simulink model "kinematic_control"  (R2018b)
settings: Solver=FixedStepAuto  StartTime=0.0  StopTime=15  FixedStep=0.001  RelTol=1e-3
values from neighbouring files (symbols this model uses):
  Cm = 0    [kinematic_parameter.m]
  Friction = 0    [kinematic_parameter.m]
  Iyw = mw*R^2/2    (= 0.0005)    [kinematic_parameter.m]
  Izb = 1/12*(d^2+w^2)    (= 0.0433333333333)    [kinematic_parameter.m]
  Izw = mw*(lx^2+ly^2)    (= 0.045487444)    [kinematic_parameter.m]
  Jm = 0    [kinematic_parameter.m]
  Kb = Kt    (= 0.0286)    [kinematic_parameter.m]
  Kf = 0    [kinematic_parameter.m]
  Ki_deg = 3    [kinematic_parameter.m]
  Ki_m = 3    [kinematic_parameter.m]
  Ki_pos = 5    [kinematic_parameter.m]
  Kp_deg = 2    [kinematic_parameter.m]
  Kp_m = 0.5    [kinematic_parameter.m]
  Kp_pos = 3    [kinematic_parameter.m]
  Kt = 28.6*10^-3    (= 0.0286)    [kinematic_parameter.m]
  La = 0.39*10^-3    (= 0.00039)    [kinematic_parameter.m]
  lx = 0.2375    [kinematic_parameter.m]
  ly = 0.2394    [kinematic_parameter.m]
  mb = 30    [kinematic_parameter.m]
  mw = 0.4    [kinematic_parameter.m]
  N = N_motor * N_wheel    (= 14)    [kinematic_parameter.m]
  R = 0.05    [kinematic_parameter.m]
  Ra = 0.38    [kinematic_parameter.m]
libraries: simulink x1
settings Model: Creator=HONG  LastModifiedBy=HONG

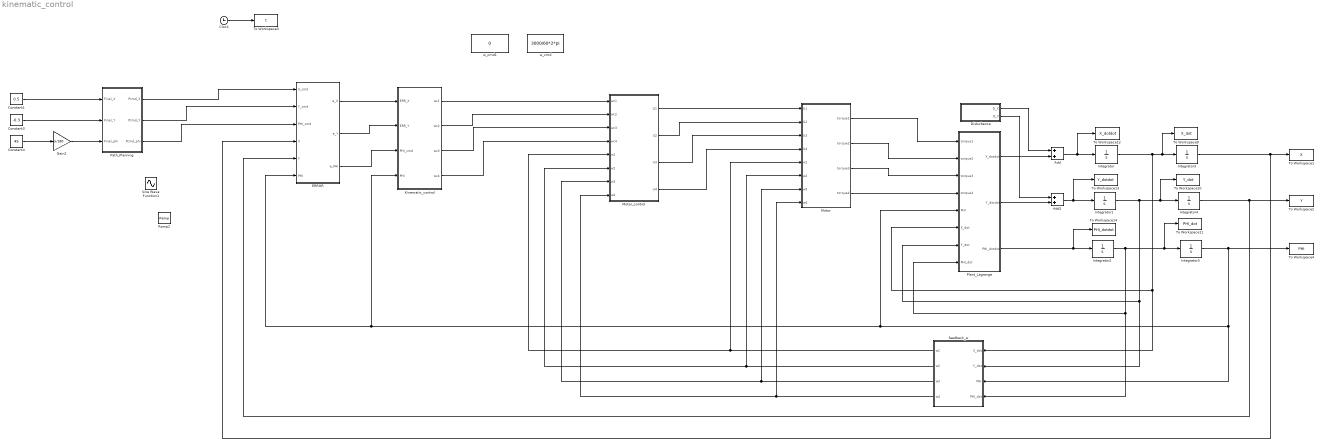
== system kinematic_control ==
  Add : Sum
  Add1 : Sum
  Clock : Clock
  Constant1 : Constant  Value=0.5
  Constant3 : Constant  Value=-0.3
  Constant4 : Constant  Value=45
  Disturbance : Subsystem
  ERROR : Subsystem
  Gain2 : Gain  Gain=pi/180
  Integrator{,1..5} (6 alike) : Integrator
  Kinematic_control : Subsystem
  Motor : Subsystem
  Motor_control : Subsystem
  Path_Planning : Subsystem
  Plant_Lagrange : Subsystem
  Ramp2 : simulink/Sources/Ramp  slope=1.2  start=0  InitialOutput=0
  Sine Wave Function1 : Sin  TimeSource=Use external signal  Frequency=pi  SampleTime=0
  To Workspace1 : ToWorkspace  VariableName=X  SampleTime=-1
  To Workspace10 : ToWorkspace  VariableName=Y_dot  SampleTime=-1
  To Workspace11 : ToWorkspace  VariableName=PHI_dot  SampleTime=-1
  To Workspace12 : ToWorkspace  VariableName=X_dotdot  SampleTime=-1
  To Workspace13 : ToWorkspace  VariableName=Y_dotdot  SampleTime=-1
  To Workspace14 : ToWorkspace  VariableName=PHI_dotdot  SampleTime=-1
  To Workspace2 : ToWorkspace  VariableName=Y  SampleTime=-1
  To Workspace3 : ToWorkspace  VariableName=t  SampleTime=-1
  To Workspace4 : ToWorkspace  VariableName=PHI  SampleTime=-1
  To Workspace9 : ToWorkspace  VariableName=X_dot  SampleTime=-1
  feedback_w : Subsystem
  w_cmd : Constant  Value=3000/60*2*pi
  w_cmd1 : Constant  Value=0
  wires:
  Integrator/1 -> To Workspace9/1, Integrator3/1, feedback_w/1(X_dot), Plant_Lagrange/6(X_dot)
  Integrator1/1 -> feedback_w/2(Y_dot), Plant_Lagrange/7(Y_dot), To Workspace10/1, Integrator4/1
  Integrator5/1 -> To Workspace4/1, feedback_w/3(PHI), ERROR/6(PHI), Kinematic_control/4(PHI), Plant_Lagrange/5(PHI)
  Integrator4/1 -> To Workspace2/1, ERROR/5(Y)
  Integrator3/1 -> ERROR/4(X), To Workspace1/1
  Plant_Lagrange/3(PHI_dotdot) -> Integrator2/1, To Workspace14/1
  Add/1 -> Integrator/1, To Workspace12/1
  Add1/1 -> Integrator1/1, To Workspace13/1
  Plant_Lagrange/1(X_dotdot) -> Add/2
  Plant_Lagrange/2(Y_dotdot) -> Add1/2
  Disturbance/2(D_Y) -> Add1/1
  Disturbance/1(D_X) -> Add/1
  Integrator2/1 -> Integrator5/1, To Workspace11/1, feedback_w/4(PHI_dot), Plant_Lagrange/8(PHI_dot)
  Clock/1 -> To Workspace3/1
  Motor/1(torque1) -> Plant_Lagrange/1("torque1 ")
  Motor/2(torque2) -> Plant_Lagrange/2("torque2 ")
  Motor/3(torque3) -> Plant_Lagrange/3(torque3)
  Motor/4(torque4) -> Plant_Lagrange/4(torque4)
  feedback_w/1(w1) -> Motor_control/5(w1), Motor/5(w1)
  feedback_w/2(w2) -> Motor_control/6(w2), Motor/6(w2)
  feedback_w/3(w3) -> Motor_control/7(w3), Motor/7(w3)
  feedback_w/4(w4) -> Motor_control/8(w4), Motor/8(w4)
  Motor_control/1(U1) -> Motor/1(U1)
  Motor_control/2(U2) -> Motor/2(U2)
  Motor_control/3(U3) -> Motor/3(U3)
  Motor_control/4(U4) -> Motor/4(U4)
  ERROR/1(e_X) -> Kinematic_control/1(ERR_X)
  ERROR/2(e_Y) -> Kinematic_control/2(ERR_Y)
  ERROR/3(e_PHI) -> Kinematic_control/3(PHI_cmd)
  Path_Planning/1(Pcmd_X) -> ERROR/1(X_cmd)
  Path_Planning/2(Pcmd_Y) -> ERROR/2(Y_cmd)
  Path_Planning/3(Pcmd_phi) -> ERROR/3(PHI_cmd)
  Kinematic_control/1(wc1) -> Motor_control/1(wc1)
  Kinematic_control/2(wc2) -> Motor_control/2(wc2)
  Kinematic_control/3(wc3) -> Motor_control/3(wc3)
  Kinematic_control/4(wc4) -> Motor_control/4(wc4)
  Constant4/1 -> Gain2/1
  Constant3/1 -> Path_Planning/2(Final_Y)
  Constant1/1 -> Path_Planning/1(Final_X)
  Gain2/1 -> Path_Planning/3(Final_phi)

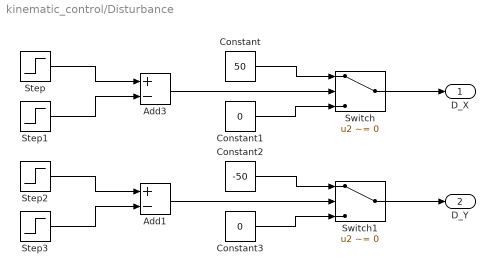
== system kinematic_control/Disturbance ==
  Add1 : Sum  Inputs=+-
  Add3 : Sum  Inputs=+-
  Constant : Constant  Value=50
  Constant1 : Constant  Value=0
  Constant2 : Constant  Value=-50
  Constant3 : Constant  Value=0
  Step{,1..3} (4 alike) : Step  Time=0  SampleTime=0
  Switch : Switch  Criteria=u2 ~= 0
  Switch1 : Switch  Criteria=u2 ~= 0
  D_X : Outport
  D_Y : Outport  Port=2
  wires:
  Add3/1 -> Switch/2
  Step1/1 -> Add3/2
  Step/1 -> Add3/1
  Constant/1 -> Switch/1
  Constant1/1 -> Switch/3
  Switch/1 -> D_X/1
  Constant2/1 -> Switch1/1
  Add1/1 -> Switch1/2
  Step2/1 -> Add1/1
  Switch1/1 -> D_Y/1
  Step3/1 -> Add1/2
  Constant3/1 -> Switch1/3

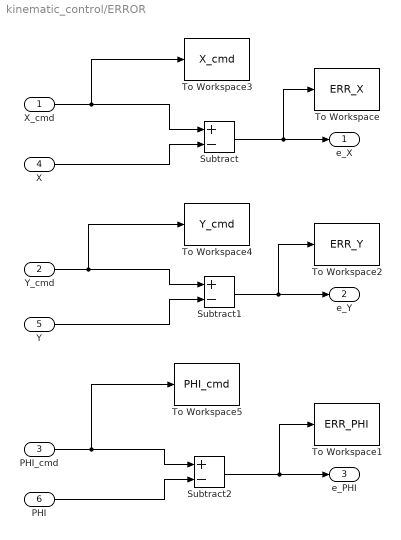
== system kinematic_control/ERROR ==
  X_cmd : Inport
  Y_cmd : Inport  Port=2
  PHI_cmd : Inport  Port=3
  X : Inport  Port=4
  Y : Inport  Port=5
  PHI : Inport  Port=6
  Subtract : Sum  Inputs=+-
  Subtract1 : Sum  Inputs=+-
  Subtract2 : Sum  Inputs=+-
  To Workspace : ToWorkspace  VariableName=ERR_X  SampleTime=-1
      settings: Save2DSignal=2-D array (concatenate along first dimension)
  To Workspace1 : ToWorkspace  VariableName=ERR_PHI  SampleTime=-1
      settings: Save2DSignal=2-D array (concatenate along first dimension)
  To Workspace2 : ToWorkspace  VariableName=ERR_Y  SampleTime=-1
      settings: Save2DSignal=2-D array (concatenate along first dimension)
  To Workspace3 : ToWorkspace  VariableName=X_cmd  SampleTime=-1
      settings: Save2DSignal=2-D array (concatenate along first dimension)
  To Workspace4 : ToWorkspace  VariableName=Y_cmd  SampleTime=-1
      settings: Save2DSignal=2-D array (concatenate along first dimension)
  To Workspace5 : ToWorkspace  VariableName=PHI_cmd  SampleTime=-1
      settings: Save2DSignal=2-D array (concatenate along first dimension)
  e_X : Outport
  e_Y : Outport  Port=2
  e_PHI : Outport  Port=3
  wires:
  X_cmd/1 -> To Workspace3/1, Subtract/1
  Subtract/1 -> To Workspace/1, e_X/1
  X/1 -> Subtract/2
  Y_cmd/1 -> To Workspace4/1, Subtract1/1
  Y/1 -> Subtract1/2
  Subtract1/1 -> To Workspace2/1, e_Y/1
  Subtract2/1 -> To Workspace1/1, e_PHI/1
  PHI_cmd/1 -> To Workspace5/1, Subtract2/1
  PHI/1 -> Subtract2/2

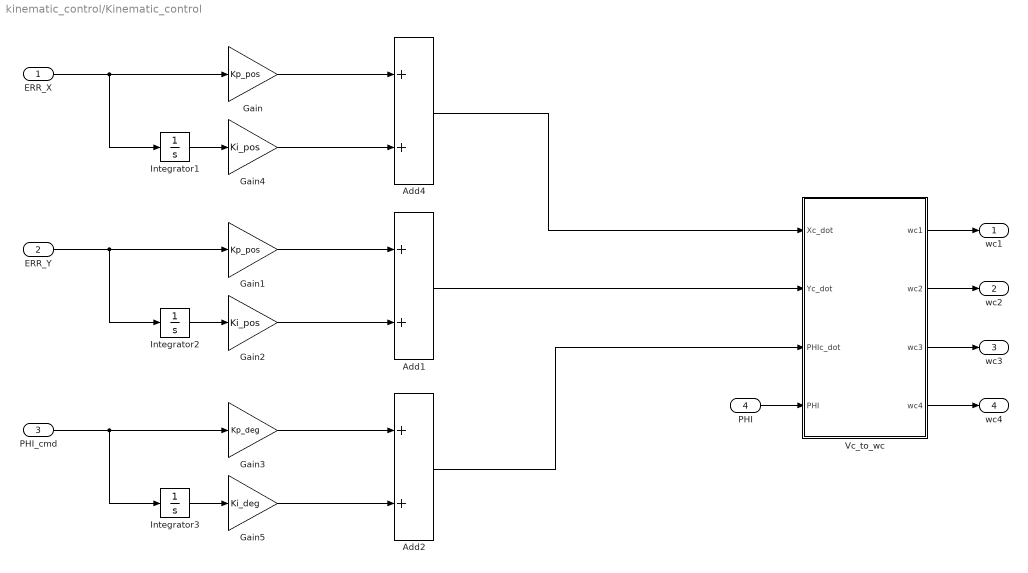
== system kinematic_control/Kinematic_control ==
  ERR_X : Inport
  ERR_Y : Inport  Port=2
  PHI_cmd : Inport  Port=3
  PHI : Inport  Port=4
  Add1 : Sum
  Add2 : Sum
  Add4 : Sum
  Gain : Gain  Gain=Kp_pos
  Gain1 : Gain  Gain=Kp_pos
  Gain2 : Gain  Gain=Ki_pos
  Gain3 : Gain  Gain=Kp_deg
  Gain4 : Gain  Gain=Ki_pos
  Gain5 : Gain  Gain=Ki_deg
  Integrator1 : Integrator
  Integrator2 : Integrator
  Integrator3 : Integrator
  Vc_to_wc : Subsystem
  wc1 : Outport
  wc2 : Outport  Port=2
  wc3 : Outport  Port=3
  wc4 : Outport  Port=4
  wires:
  Vc_to_wc/1(wc1) -> wc1/1
  Vc_to_wc/2(wc2) -> wc2/1
  Vc_to_wc/3(wc3) -> wc3/1
  Vc_to_wc/4(wc4) -> wc4/1
  Gain/1 -> Add4/1
  ERR_X/1 -> Gain/1, Integrator1/1
  Integrator1/1 -> Gain4/1
  Gain4/1 -> Add4/2
  PHI/1 -> Vc_to_wc/4(PHI)
  Gain1/1 -> Add1/1
  Gain2/1 -> Add1/2
  ERR_Y/1 -> Gain1/1, Integrator2/1
  Integrator2/1 -> Gain2/1
  Integrator3/1 -> Gain5/1
  Gain3/1 -> Add2/1
  Gain5/1 -> Add2/2
  PHI_cmd/1 -> Gain3/1, Integrator3/1
  Add4/1 -> Vc_to_wc/1(Xc_dot)
  Add1/1 -> Vc_to_wc/2(Yc_dot)
  Add2/1 -> Vc_to_wc/3(PHIc_dot)

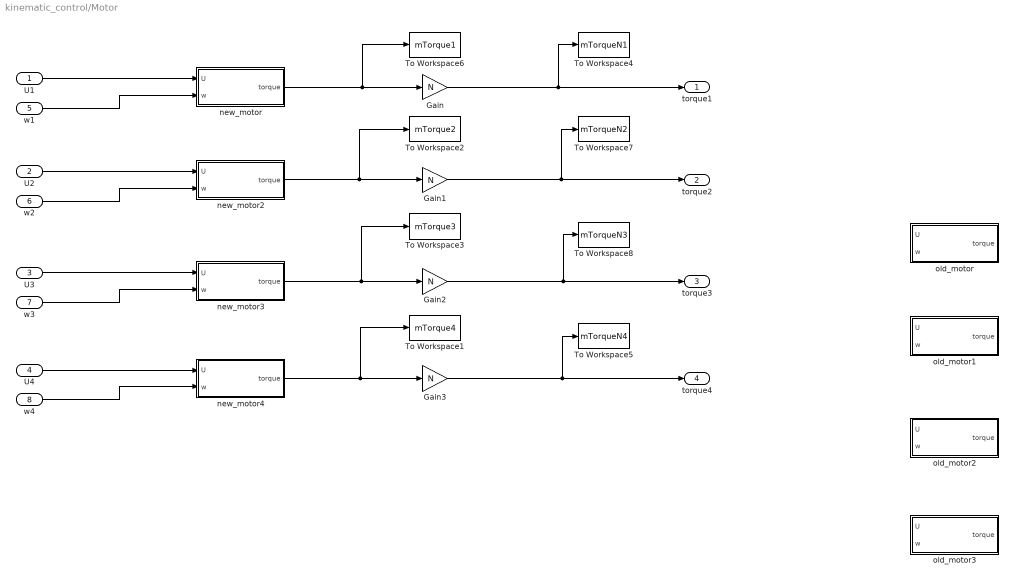
== system kinematic_control/Motor ==
  U1 : Inport
  U2 : Inport  Port=2
  U3 : Inport  Port=3
  U4 : Inport  Port=4
  w1 : Inport  Port=5
  w2 : Inport  Port=6
  w3 : Inport  Port=7
  w4 : Inport  Port=8
  Gain{,1..3} (4 alike) : Gain  Gain=N
  To Workspace1 : ToWorkspace  VariableName=mTorque4  SampleTime=-1
  To Workspace2 : ToWorkspace  VariableName=mTorque2  SampleTime=-1
  To Workspace3 : ToWorkspace  VariableName=mTorque3  SampleTime=-1
  To Workspace4 : ToWorkspace  VariableName=mTorqueN1  SampleTime=-1
  To Workspace5 : ToWorkspace  VariableName=mTorqueN4  SampleTime=-1
  To Workspace6 : ToWorkspace  VariableName=mTorque1  SampleTime=-1
  To Workspace7 : ToWorkspace  VariableName=mTorqueN2  SampleTime=-1
  To Workspace8 : ToWorkspace  VariableName=mTorqueN3  SampleTime=-1
  new_motor : Subsystem
  new_motor2 : Subsystem
  new_motor3 : Subsystem
  new_motor4 : Subsystem
  old_motor : Subsystem
  old_motor1 : Subsystem
  old_motor2 : Subsystem
  old_motor3 : Subsystem
  torque1 : Outport
  torque2 : Outport  Port=2
  torque3 : Outport  Port=3
  torque4 : Outport  Port=4
  wires:
  U1/1 -> new_motor/1(U)
  w1/1 -> new_motor/2(w)
  w2/1 -> new_motor2/2(w)
  U2/1 -> new_motor2/1(U)
  U3/1 -> new_motor3/1(U)
  w3/1 -> new_motor3/2(w)
  U4/1 -> new_motor4/1(U)
  w4/1 -> new_motor4/2(w)
  new_motor/1(torque) -> To Workspace6/1, Gain/1
  new_motor2/1(torque) -> To Workspace2/1, Gain1/1
  new_motor3/1(torque) -> To Workspace3/1, Gain2/1
  new_motor4/1(torque) -> Gain3/1, To Workspace1/1
  Gain1/1 -> To Workspace7/1, torque2/1
  Gain2/1 -> To Workspace8/1, torque3/1
  Gain3/1 -> To Workspace5/1, torque4/1
  Gain/1 -> To Workspace4/1, torque1/1

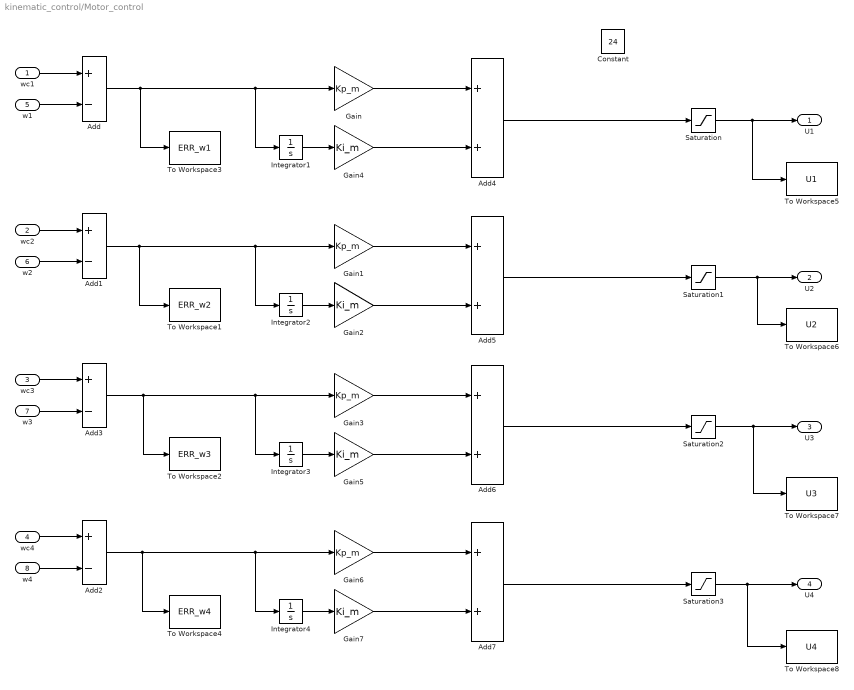
== system kinematic_control/Motor_control ==
  wc1 : Inport
  wc2 : Inport  Port=2
  wc3 : Inport  Port=3
  wc4 : Inport  Port=4
  w1 : Inport  Port=5
  w2 : Inport  Port=6
  w3 : Inport  Port=7
  w4 : Inport  Port=8
  Add{,1..3} (4 alike) : Sum  Inputs=+-
  Add{4..7} (4 alike) : Sum
  Constant : Constant  Value=24
  Gain{,1,3,6} (4 alike) : Gain  Gain=Kp_m
  Gain{2,4..5,7} (4 alike) : Gain  Gain=Ki_m
  Integrator{1..4} (4 alike) : Integrator
  Saturation{,1..3} (4 alike) : Saturate  UpperLimit=24  LowerLimit=-24
  To Workspace1 : ToWorkspace  VariableName=ERR_w2  SampleTime=-1
      settings: Save2DSignal=2-D array (concatenate along first dimension)
  To Workspace2 : ToWorkspace  VariableName=ERR_w3  SampleTime=-1
      settings: Save2DSignal=2-D array (concatenate along first dimension)
  To Workspace3 : ToWorkspace  VariableName=ERR_w1  SampleTime=-1
      settings: Save2DSignal=2-D array (concatenate along first dimension)
  To Workspace4 : ToWorkspace  VariableName=ERR_w4  SampleTime=-1
      settings: Save2DSignal=2-D array (concatenate along first dimension)
  To Workspace5 : ToWorkspace  VariableName=U1  SampleTime=-1
      settings: Save2DSignal=2-D array (concatenate along first dimension)
  To Workspace6 : ToWorkspace  VariableName=U2  SampleTime=-1
      settings: Save2DSignal=2-D array (concatenate along first dimension)
  To Workspace7 : ToWorkspace  VariableName=U3  SampleTime=-1
      settings: Save2DSignal=2-D array (concatenate along first dimension)
  To Workspace8 : ToWorkspace  VariableName=U4  SampleTime=-1
      settings: Save2DSignal=2-D array (concatenate along first dimension)
  U1 : Outport
  U2 : Outport  Port=2
  U3 : Outport  Port=3
  U4 : Outport  Port=4
  wires:
  wc1/1 -> Add/1
  w1/1 -> Add/2
  w4/1 -> Add2/2
  w3/1 -> Add3/2
  wc3/1 -> Add3/1
  w2/1 -> Add1/2
  wc2/1 -> Add1/1
  wc4/1 -> Add2/1
  Add/1 -> Integrator1/1, Gain/1, To Workspace3/1
  Integrator1/1 -> Gain4/1
  Integrator2/1 -> Gain2/1
  Add1/1 -> To Workspace1/1, Integrator2/1, Gain1/1
  Integrator3/1 -> Gain5/1
  Add3/1 -> To Workspace2/1, Integrator3/1, Gain3/1
  Integrator4/1 -> Gain7/1
  Add2/1 -> To Workspace4/1, Integrator4/1, Gain6/1
  Gain/1 -> Add4/1
  Gain4/1 -> Add4/2
  Gain1/1 -> Add5/1
  Gain2/1 -> Add5/2
  Gain3/1 -> Add6/1
  Gain5/1 -> Add6/2
  Gain6/1 -> Add7/1
  Gain7/1 -> Add7/2
  Saturation/1 -> To Workspace5/1, U1/1
  Saturation3/1 -> To Workspace8/1, U4/1
  Saturation2/1 -> To Workspace7/1, U3/1
  Saturation1/1 -> To Workspace6/1, U2/1
  Add4/1 -> Saturation/1
  Add5/1 -> Saturation1/1
  Add6/1 -> Saturation2/1
  Add7/1 -> Saturation3/1

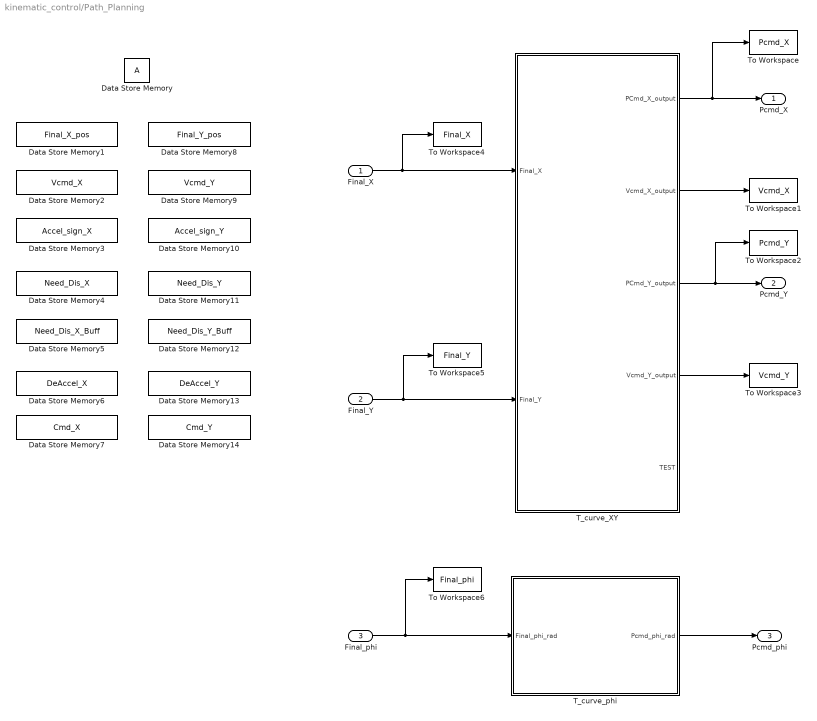
== system kinematic_control/Path_Planning ==
  Final_X : Inport
  Final_Y : Inport  Port=2
  Final_phi : Inport  Port=3
  Data Store Memory : DataStoreMemory  ReadBeforeWriteMsg=warning  WriteAfterWriteMsg=warning  WriteAfterReadMsg=warning  ShowAdditionalParam=off  OutDataTypeStr=double
  Data Store Memory1 : DataStoreMemory  DataStoreName=Final_X_pos  ReadBeforeWriteMsg=warning  WriteAfterWriteMsg=warning  WriteAfterReadMsg=warning  ShowAdditionalParam=off  OutDataTypeStr=double
  Data Store Memory10 : DataStoreMemory  DataStoreName=Accel_sign_Y  ReadBeforeWriteMsg=warning  WriteAfterWriteMsg=warning  WriteAfterReadMsg=warning  ShowAdditionalParam=off  OutDataTypeStr=double
  Data Store Memory11 : DataStoreMemory  DataStoreName=Need_Dis_Y  ReadBeforeWriteMsg=warning  WriteAfterWriteMsg=warning  WriteAfterReadMsg=warning  ShowAdditionalParam=off  OutDataTypeStr=double
  Data Store Memory12 : DataStoreMemory  DataStoreName=Need_Dis_Y_Buff  ReadBeforeWriteMsg=warning  WriteAfterWriteMsg=warning  WriteAfterReadMsg=warning  ShowAdditionalParam=off  OutDataTypeStr=double
  Data Store Memory13 : DataStoreMemory  DataStoreName=DeAccel_Y  ReadBeforeWriteMsg=warning  WriteAfterWriteMsg=warning  WriteAfterReadMsg=warning  ShowAdditionalParam=off  OutDataTypeStr=double
  Data Store Memory14 : DataStoreMemory  DataStoreName=Cmd_Y  ReadBeforeWriteMsg=warning  WriteAfterWriteMsg=warning  WriteAfterReadMsg=warning  ShowAdditionalParam=off  OutDataTypeStr=double
  Data Store Memory2 : DataStoreMemory  DataStoreName=Vcmd_X  ReadBeforeWriteMsg=warning  WriteAfterWriteMsg=warning  WriteAfterReadMsg=warning  ShowAdditionalParam=off  OutDataTypeStr=double
  Data Store Memory3 : DataStoreMemory  DataStoreName=Accel_sign_X  ReadBeforeWriteMsg=warning  WriteAfterWriteMsg=warning  WriteAfterReadMsg=warning  ShowAdditionalParam=off  OutDataTypeStr=double
  Data Store Memory4 : DataStoreMemory  DataStoreName=Need_Dis_X  ReadBeforeWriteMsg=warning  WriteAfterWriteMsg=warning  WriteAfterReadMsg=warning  ShowAdditionalParam=off  OutDataTypeStr=double
  Data Store Memory5 : DataStoreMemory  DataStoreName=Need_Dis_X_Buff  ReadBeforeWriteMsg=warning  WriteAfterWriteMsg=warning  WriteAfterReadMsg=warning  ShowAdditionalParam=off  OutDataTypeStr=double
  Data Store Memory6 : DataStoreMemory  DataStoreName=DeAccel_X  ReadBeforeWriteMsg=warning  WriteAfterWriteMsg=warning  WriteAfterReadMsg=warning  ShowAdditionalParam=off  OutDataTypeStr=double
  Data Store Memory7 : DataStoreMemory  DataStoreName=Cmd_X  ReadBeforeWriteMsg=warning  WriteAfterWriteMsg=warning  WriteAfterReadMsg=warning  ShowAdditionalParam=off  OutDataTypeStr=double
  Data Store Memory8 : DataStoreMemory  DataStoreName=Final_Y_pos  ReadBeforeWriteMsg=warning  WriteAfterWriteMsg=warning  WriteAfterReadMsg=warning  ShowAdditionalParam=off  OutDataTypeStr=double
  Data Store Memory9 : DataStoreMemory  DataStoreName=Vcmd_Y  ReadBeforeWriteMsg=warning  WriteAfterWriteMsg=warning  WriteAfterReadMsg=warning  ShowAdditionalParam=off  OutDataTypeStr=double
  "T_curve_XY " : MATLAB Function  TreatAsAtomicUnit=on
  T_curve_phi : Subsystem
  To Workspace : ToWorkspace  VariableName=Pcmd_X  SampleTime=-1
  To Workspace1 : ToWorkspace  VariableName=Vcmd_X  SampleTime=-1
  To Workspace2 : ToWorkspace  VariableName=Pcmd_Y  SampleTime=-1
  To Workspace3 : ToWorkspace  VariableName=Vcmd_Y  SampleTime=-1
  To Workspace4 : ToWorkspace  VariableName=Final_X  SampleTime=-1
  To Workspace5 : ToWorkspace  VariableName=Final_Y  SampleTime=-1
  To Workspace6 : ToWorkspace  VariableName=Final_phi  SampleTime=-1
  Pcmd_X : Outport
  Pcmd_Y : Outport  Port=2
  Pcmd_phi : Outport  Port=3
  wires:
  Final_X/1 -> To Workspace4/1, "T_curve_XY "/1(Final_X)
  Final_Y/1 -> To Workspace5/1, "T_curve_XY "/2(Final_Y)
  "T_curve_XY "/1(PCmd_X_output) -> To Workspace/1, Pcmd_X/1
  "T_curve_XY "/3(PCmd_Y_output) -> To Workspace2/1, Pcmd_Y/1
  "T_curve_XY "/2(Vcmd_X_output) -> To Workspace1/1
  "T_curve_XY "/4(Vcmd_Y_output) -> To Workspace3/1
  Final_phi/1 -> To Workspace6/1, T_curve_phi/1(Final_phi_rad)
  T_curve_phi/1(Pcmd_phi_rad) -> Pcmd_phi/1

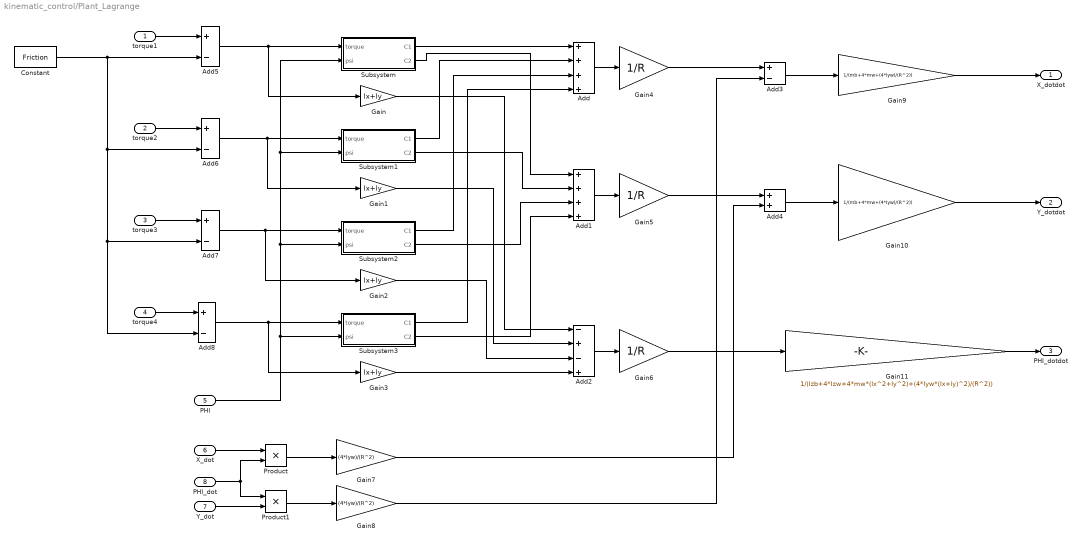
== system kinematic_control/Plant_Lagrange ==
  "torque1 " : Inport
  "torque2 " : Inport  Port=2
  torque3 : Inport  Port=3
  torque4 : Inport  Port=4
  PHI : Inport  Port=5
  X_dot : Inport  Port=6
  Y_dot : Inport  Port=7
  PHI_dot : Inport  Port=8
  Add : Sum  Inputs=++++
  Add1 : Sum  Inputs=++++
  Add2 : Sum  Inputs=-+-+
  Add{3,5..8} (5 alike) : Sum  Inputs=+-
  Add4 : Sum
  Constant : Constant  Value=Friction
  Gain{,1..3} (4 alike) : Gain  Gain=lx+ly
  Gain10 : Gain  Gain=1/(mb+4*mw+(4*Iyw)/(R^2))
  Gain11 : Gain  Gain=1/(Izb+4*Izw+4*mw*(lx^2+ly^2)+(4*Iyw*(lx+ly)^2)/(R^2))
  Gain4 : Gain  Gain=1/R
  Gain5 : Gain  Gain=1/R
  Gain6 : Gain  Gain=1/R
  Gain7 : Gain  Gain=(4*Iyw)/(R^2)
  Gain8 : Gain  Gain=(4*Iyw)/(R^2)
  Gain9 : Gain  Gain=1/(mb+4*mw+(4*Iyw)/(R^2))
  Product : Product
  Product1 : Product
  Subsystem : Subsystem
  Subsystem1 : Subsystem
  Subsystem2 : Subsystem
  Subsystem3 : Subsystem
  X_dotdot : Outport
  Y_dotdot : Outport  Port=2
  PHI_dotdot : Outport  Port=3
  wires:
  Add7/1 -> Gain2/1, Subsystem2/1(torque)
  Add8/1 -> Gain3/1, Subsystem3/1(torque)
  PHI/1 -> Subsystem3/2("psi "), Subsystem2/2("psi "), Subsystem1/2("psi "), Subsystem/2("psi ")
  Add6/1 -> Gain1/1, Subsystem1/1(torque)
  Subsystem/1(C1) -> Add/1
  Subsystem1/1(C1) -> Add/2
  Subsystem2/1(C1) -> Add/3
  Subsystem3/1(C1) -> Add/4
  Subsystem/2(C2) -> Add1/1
  Subsystem1/2(C2) -> Add1/2
  Subsystem2/2(C2) -> Add1/3
  Subsystem3/2(C2) -> Add1/4
  Gain/1 -> Add2/1
  Gain1/1 -> Add2/2
  Gain2/1 -> Add2/3
  Gain3/1 -> Add2/4
  Add1/1 -> Gain5/1
  Add/1 -> Gain4/1
  Add2/1 -> Gain6/1
  Y_dot/1 -> Product1/2
  PHI_dot/1 -> Product/2, Product1/1
  X_dot/1 -> Product/1
  Product/1 -> Gain7/1
  Product1/1 -> Gain8/1
  Gain4/1 -> Add3/1
  Gain5/1 -> Add4/1
  Gain8/1 -> Add3/2
  Gain7/1 -> Add4/2
  Add3/1 -> Gain9/1
  Add4/1 -> Gain10/1
  Gain6/1 -> Gain11/1
  Gain9/1 -> X_dotdot/1
  Gain10/1 -> Y_dotdot/1
  Gain11/1 -> PHI_dotdot/1
  Add5/1 -> Gain/1, Subsystem/1(torque)
  "torque1 "/1 -> Add5/1
  Constant/1 -> Add7/2, Add8/2, Add6/2, Add5/2
  "torque2 "/1 -> Add6/1
  torque3/1 -> Add7/1
  torque4/1 -> Add8/1

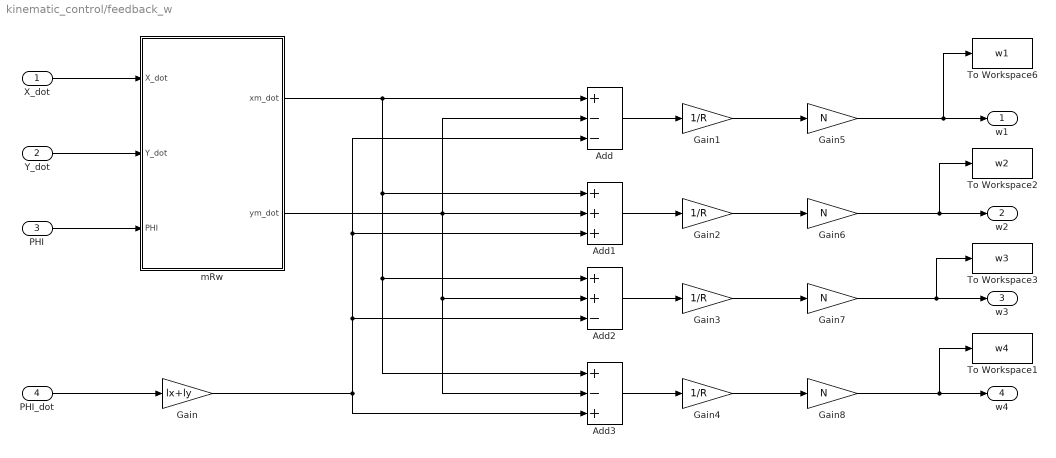
== system kinematic_control/feedback_w ==
  X_dot : Inport
  Y_dot : Inport  Port=2
  PHI : Inport  Port=3
  PHI_dot : Inport  Port=4
  Add : Sum  Inputs=+--
  Add1 : Sum  Inputs=+++
  Add2 : Sum  Inputs=++-
  Add3 : Sum  Inputs=+-+
  Gain : Gain  Gain=lx+ly
  Gain{1..4} (4 alike) : Gain  Gain=1/R
  Gain{5..8} (4 alike) : Gain  Gain=N
  To Workspace1 : ToWorkspace  VariableName=w4  SampleTime=-1
  To Workspace2 : ToWorkspace  VariableName=w2  SampleTime=-1
  To Workspace3 : ToWorkspace  VariableName=w3  SampleTime=-1
  To Workspace6 : ToWorkspace  VariableName=w1  SampleTime=-1
  mRw : Subsystem
  w1 : Outport
  w2 : Outport  Port=2
  w3 : Outport  Port=3
  w4 : Outport  Port=4
  wires:
  Y_dot/1 -> mRw/2(Y_dot)
  PHI/1 -> mRw/3(PHI)
  PHI_dot/1 -> Gain/1
  mRw/1(xm_dot) -> Add3/1, Add2/1, Add1/1, Add/1
  Add/1 -> Gain1/1
  Add1/1 -> Gain2/1
  Add2/1 -> Gain3/1
  Add3/1 -> Gain4/1
  mRw/2(ym_dot) -> Add3/2, Add2/2, Add1/2, Add/2
  Gain/1 -> Add2/3, Add1/3, Add/3, Add3/3
  Gain1/1 -> Gain5/1
  Gain2/1 -> Gain6/1
  Gain3/1 -> Gain7/1
  Gain4/1 -> Gain8/1
  X_dot/1 -> mRw/1(X_dot)
  Gain5/1 -> w1/1, To Workspace6/1
  Gain6/1 -> w2/1, To Workspace2/1
  Gain7/1 -> To Workspace3/1, w3/1
  Gain8/1 -> To Workspace1/1, w4/1

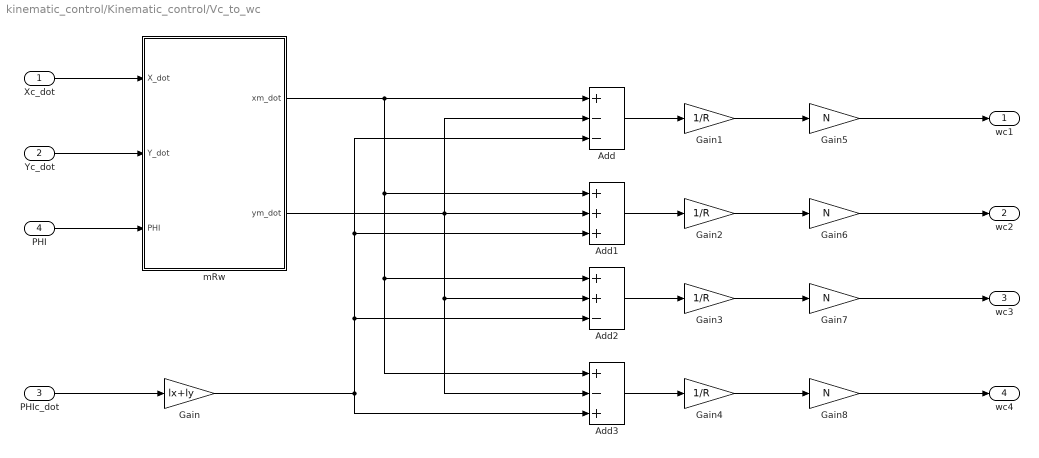
== system kinematic_control/Kinematic_control/Vc_to_wc ==
  Xc_dot : Inport
  Yc_dot : Inport  Port=2
  PHIc_dot : Inport  Port=3
  PHI : Inport  Port=4
  Add : Sum  Inputs=+--
  Add1 : Sum  Inputs=+++
  Add2 : Sum  Inputs=++-
  Add3 : Sum  Inputs=+-+
  Gain : Gain  Gain=lx+ly
  Gain{1..4} (4 alike) : Gain  Gain=1/R
  Gain{5..8} (4 alike) : Gain  Gain=N
  mRw : Subsystem
  wc1 : Outport
  wc2 : Outport  Port=2
  wc3 : Outport  Port=3
  wc4 : Outport  Port=4
  wires:
  Yc_dot/1 -> mRw/2(Y_dot)
  PHI/1 -> mRw/3(PHI)
  PHIc_dot/1 -> Gain/1
  mRw/1(xm_dot) -> Add3/1, Add2/1, Add1/1, Add/1
  Add/1 -> Gain1/1
  Add1/1 -> Gain2/1
  Add2/1 -> Gain3/1
  Add3/1 -> Gain4/1
  mRw/2(ym_dot) -> Add3/2, Add2/2, Add1/2, Add/2
  Gain/1 -> Add2/3, Add1/3, Add/3, Add3/3
  Gain1/1 -> Gain5/1
  Gain2/1 -> Gain6/1
  Gain3/1 -> Gain7/1
  Gain4/1 -> Gain8/1
  Xc_dot/1 -> mRw/1(X_dot)
  Gain5/1 -> wc1/1
  Gain6/1 -> wc2/1
  Gain7/1 -> wc3/1
  Gain8/1 -> wc4/1

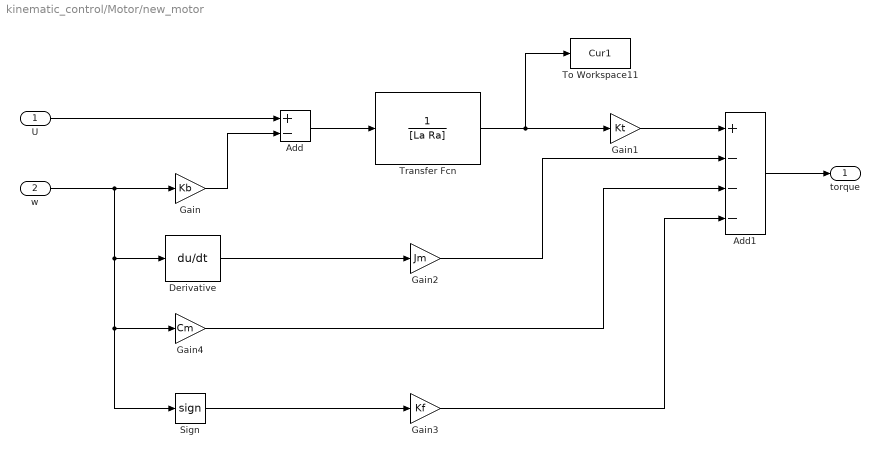
== system kinematic_control/Motor/new_motor ==
  U : Inport
  w : Inport  Port=2
  Add : Sum  Inputs=+-
  Add1 : Sum  Inputs=+---
  Derivative : Derivative
  Gain : Gain  Gain=Kb
  Gain1 : Gain  Gain=Kt
  Gain2 : Gain  Gain=Jm
  Gain3 : Gain  Gain=Kf
  Gain4 : Gain  Gain=Cm
  Sign : Signum  ZeroCross=off
  To Workspace11 : ToWorkspace  VariableName=Cur1  SampleTime=-1
  Transfer Fcn : TransferFcn  Denominator=[La Ra]
  torque : Outport
  wires:
  Add1/1 -> torque/1
  Gain2/1 -> Add1/2
  Derivative/1 -> Gain2/1
  Gain1/1 -> Add1/1
  Gain4/1 -> Add1/3
  Add/1 -> Transfer Fcn/1
  Gain/1 -> Add/2
  Transfer Fcn/1 -> To Workspace11/1, Gain1/1
  Sign/1 -> Gain3/1
  w/1 -> Sign/1, Gain4/1, Derivative/1, Gain/1
  U/1 -> Add/1
  Gain3/1 -> Add1/4

== system kinematic_control/Motor/new_motor2 ==
  U : Inport
  w : Inport  Port=2
  Add : Sum  Inputs=+-
  Add1 : Sum  Inputs=+---
  Derivative : Derivative
  Gain : Gain  Gain=Kb
  Gain1 : Gain  Gain=Kt
  Gain2 : Gain  Gain=Jm
  Gain3 : Gain  Gain=Kf
  Gain4 : Gain  Gain=Cm
  Sign : Signum  ZeroCross=off
  To Workspace11 : ToWorkspace  VariableName=Cur2  SampleTime=-1
  Transfer Fcn : TransferFcn  Denominator=[La Ra]
  torque : Outport
  wires:
  Add1/1 -> torque/1
  Gain2/1 -> Add1/2
  Derivative/1 -> Gain2/1
  Gain1/1 -> Add1/1
  Gain4/1 -> Add1/3
  Add/1 -> Transfer Fcn/1
  Gain/1 -> Add/2
  Transfer Fcn/1 -> To Workspace11/1, Gain1/1
  Sign/1 -> Gain3/1
  w/1 -> Sign/1, Gain4/1, Derivative/1, Gain/1
  U/1 -> Add/1
  Gain3/1 -> Add1/4

== system kinematic_control/Motor/new_motor3 ==
  U : Inport
  w : Inport  Port=2
  Add : Sum  Inputs=+-
  Add1 : Sum  Inputs=+---
  Derivative : Derivative
  Gain : Gain  Gain=Kb
  Gain1 : Gain  Gain=Kt
  Gain2 : Gain  Gain=Jm
  Gain3 : Gain  Gain=Kf
  Gain4 : Gain  Gain=Cm
  Sign : Signum  ZeroCross=off
  To Workspace11 : ToWorkspace  VariableName=Cur3  SampleTime=-1
  Transfer Fcn : TransferFcn  Denominator=[La Ra]
  torque : Outport
  wires:
  Add1/1 -> torque/1
  Gain2/1 -> Add1/2
  Derivative/1 -> Gain2/1
  Gain1/1 -> Add1/1
  Gain4/1 -> Add1/3
  Add/1 -> Transfer Fcn/1
  Gain/1 -> Add/2
  Transfer Fcn/1 -> To Workspace11/1, Gain1/1
  Sign/1 -> Gain3/1
  w/1 -> Sign/1, Gain4/1, Derivative/1, Gain/1
  U/1 -> Add/1
  Gain3/1 -> Add1/4

== system kinematic_control/Motor/new_motor4 ==
  U : Inport
  w : Inport  Port=2
  Add : Sum  Inputs=+-
  Add1 : Sum  Inputs=+---
  Derivative : Derivative
  Gain : Gain  Gain=Kb
  Gain1 : Gain  Gain=Kt
  Gain2 : Gain  Gain=Jm
  Gain3 : Gain  Gain=Kf
  Gain4 : Gain  Gain=Cm
  Sign : Signum  ZeroCross=off
  To Workspace11 : ToWorkspace  VariableName=Cur4  SampleTime=-1
  Transfer Fcn : TransferFcn  Denominator=[La Ra]
  torque : Outport
  wires:
  Add1/1 -> torque/1
  Gain2/1 -> Add1/2
  Derivative/1 -> Gain2/1
  Gain1/1 -> Add1/1
  Gain4/1 -> Add1/3
  Add/1 -> Transfer Fcn/1
  Gain/1 -> Add/2
  Transfer Fcn/1 -> To Workspace11/1, Gain1/1
  Sign/1 -> Gain3/1
  w/1 -> Sign/1, Gain4/1, Derivative/1, Gain/1
  U/1 -> Add/1
  Gain3/1 -> Add1/4

== system kinematic_control/Motor/old_motor ==
  U : Inport
  w : Inport  Port=2
  Add : Sum  Inputs=+-
  Gain : Gain  Gain=Kb*Kb/Ra
  Gain1 : Gain  Gain=Kb/Ra
  torque : Outport
  wires:
  U/1 -> Gain1/1
  w/1 -> Gain/1
  Gain1/1 -> Add/1
  Gain/1 -> Add/2
  Add/1 -> torque/1

== system kinematic_control/Motor/old_motor1 ==
  U : Inport
  w : Inport  Port=2
  Add : Sum  Inputs=+-
  Gain : Gain  Gain=Kb*Kb/Ra
  Gain1 : Gain  Gain=Kb/Ra
  torque : Outport
  wires:
  U/1 -> Gain1/1
  w/1 -> Gain/1
  Gain1/1 -> Add/1
  Gain/1 -> Add/2
  Add/1 -> torque/1

== system kinematic_control/Motor/old_motor2 ==
  U : Inport
  w : Inport  Port=2
  Add : Sum  Inputs=+-
  Gain : Gain  Gain=Kb*Kb/Ra
  Gain1 : Gain  Gain=Kb/Ra
  torque : Outport
  wires:
  U/1 -> Gain1/1
  w/1 -> Gain/1
  Gain1/1 -> Add/1
  Gain/1 -> Add/2
  Add/1 -> torque/1

== system kinematic_control/Motor/old_motor3 ==
  U : Inport
  w : Inport  Port=2
  Add : Sum  Inputs=+-
  Gain : Gain  Gain=Kb*Kb/Ra
  Gain1 : Gain  Gain=Kb/Ra
  torque : Outport
  wires:
  U/1 -> Gain1/1
  w/1 -> Gain/1
  Gain1/1 -> Add/1
  Gain/1 -> Add/2
  Add/1 -> torque/1

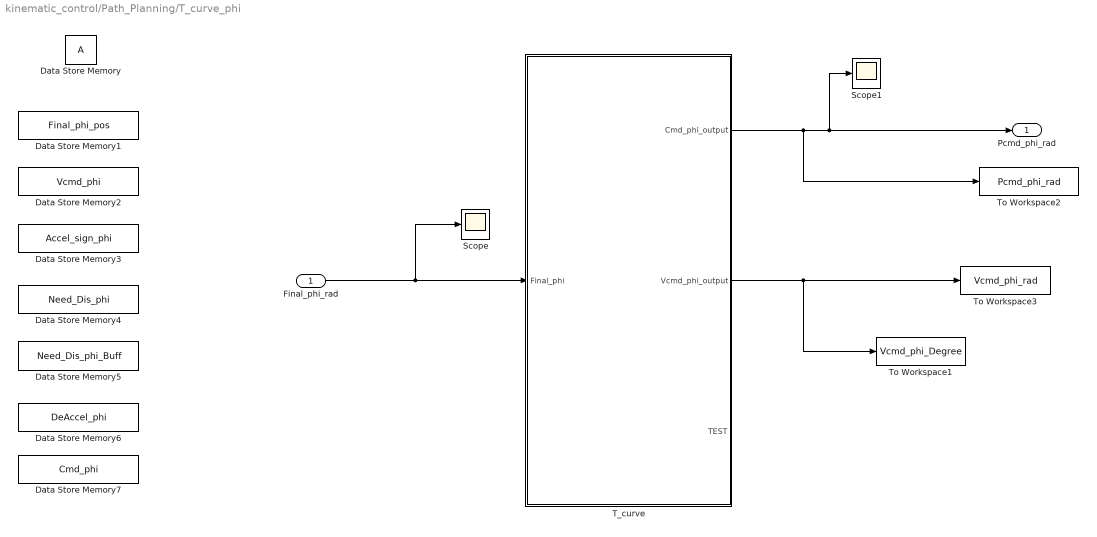
== system kinematic_control/Path_Planning/T_curve_phi ==
  Final_phi_rad : Inport
  Data Store Memory : DataStoreMemory  ReadBeforeWriteMsg=warning  WriteAfterWriteMsg=warning  WriteAfterReadMsg=warning  ShowAdditionalParam=off  OutDataTypeStr=double
  Data Store Memory1 : DataStoreMemory  DataStoreName=Final_phi_pos  ReadBeforeWriteMsg=warning  WriteAfterWriteMsg=warning  WriteAfterReadMsg=warning  ShowAdditionalParam=off  OutDataTypeStr=double
  Data Store Memory2 : DataStoreMemory  DataStoreName=Vcmd_phi  ReadBeforeWriteMsg=warning  WriteAfterWriteMsg=warning  WriteAfterReadMsg=warning  ShowAdditionalParam=off  OutDataTypeStr=double
  Data Store Memory3 : DataStoreMemory  DataStoreName=Accel_sign_phi  ReadBeforeWriteMsg=warning  WriteAfterWriteMsg=warning  WriteAfterReadMsg=warning  ShowAdditionalParam=off  OutDataTypeStr=double
  Data Store Memory4 : DataStoreMemory  DataStoreName=Need_Dis_phi  ReadBeforeWriteMsg=warning  WriteAfterWriteMsg=warning  WriteAfterReadMsg=warning  ShowAdditionalParam=off  OutDataTypeStr=double
  Data Store Memory5 : DataStoreMemory  DataStoreName=Need_Dis_phi_Buff  ReadBeforeWriteMsg=warning  WriteAfterWriteMsg=warning  WriteAfterReadMsg=warning  ShowAdditionalParam=off  OutDataTypeStr=double
  Data Store Memory6 : DataStoreMemory  DataStoreName=DeAccel_phi  ReadBeforeWriteMsg=warning  WriteAfterWriteMsg=warning  WriteAfterReadMsg=warning  ShowAdditionalParam=off  OutDataTypeStr=double
  Data Store Memory7 : DataStoreMemory  DataStoreName=Cmd_phi  ReadBeforeWriteMsg=warning  WriteAfterWriteMsg=warning  WriteAfterReadMsg=warning  ShowAdditionalParam=off  OutDataTypeStr=double
  Scope : Scope
  Scope1 : Scope
  T_curve : MATLAB Function  TreatAsAtomicUnit=on
  To Workspace1 : ToWorkspace  VariableName=Vcmd_phi_Degree  SampleTime=-1
  To Workspace2 : ToWorkspace  VariableName=Pcmd_phi_rad  SampleTime=-1
  To Workspace3 : ToWorkspace  VariableName=Vcmd_phi_rad  SampleTime=-1
  Pcmd_phi_rad : Outport
  wires:
  Final_phi_rad/1 -> T_curve/1(Final_phi), Scope/1
  T_curve/2(Vcmd_phi_output) -> To Workspace3/1, To Workspace1/1
  T_curve/1(Cmd_phi_output) -> Scope1/1, Pcmd_phi_rad/1, To Workspace2/1

== system kinematic_control/Plant_Lagrange/Subsystem ==
  torque : Inport
  "psi " : Inport  Port=2
  -C+S : Sum  Inputs=-+
  C+S : Sum
  Product : Product
  Product1 : Product
  Trigonometric Function : Trigonometry
  Trigonometric Function1 : Trigonometry  Operator=cos
  C1 : Outport
  C2 : Outport  Port=2
  wires:
  Trigonometric Function/1 -> -C+S/2, C+S/2
  Trigonometric Function1/1 -> C+S/1, -C+S/1
  "psi "/1 -> Trigonometric Function/1, Trigonometric Function1/1
  torque/1 -> Product1/1, Product/1
  C+S/1 -> Product/2
  Product/1 -> C1/1
  Product1/1 -> C2/1
  -C+S/1 -> Product1/2

== system kinematic_control/Plant_Lagrange/Subsystem1 ==
  torque : Inport
  "psi " : Inport  Port=2
  C+S : Sum
  C-S : Sum  Inputs=+-
  Product : Product
  Product1 : Product
  Trigonometric Function : Trigonometry
  Trigonometric Function1 : Trigonometry  Operator=cos
  C1 : Outport
  C2 : Outport  Port=2
  wires:
  Trigonometric Function/1 -> C-S/2, C+S/2
  Trigonometric Function1/1 -> C+S/1, C-S/1
  "psi "/1 -> Trigonometric Function/1, Trigonometric Function1/1
  torque/1 -> Product1/1, Product/1
  Product/1 -> C1/1
  Product1/1 -> C2/1
  C-S/1 -> Product/2
  C+S/1 -> Product1/2

== system kinematic_control/Plant_Lagrange/Subsystem2 ==
  torque : Inport
  "psi " : Inport  Port=2
  C+S : Sum
  C-S : Sum  Inputs=+-
  Product : Product
  Product1 : Product
  Trigonometric Function : Trigonometry
  Trigonometric Function1 : Trigonometry  Operator=cos
  C1 : Outport
  C2 : Outport  Port=2
  wires:
  Trigonometric Function/1 -> C-S/2, C+S/2
  Trigonometric Function1/1 -> C+S/1, C-S/1
  "psi "/1 -> Trigonometric Function/1, Trigonometric Function1/1
  torque/1 -> Product1/1, Product/1
  Product/1 -> C1/1
  Product1/1 -> C2/1
  C-S/1 -> Product/2
  C+S/1 -> Product1/2

== system kinematic_control/Plant_Lagrange/Subsystem3 ==
  torque : Inport
  "psi " : Inport  Port=2
  -C+S : Sum  Inputs=-+
  C+S : Sum
  Product : Product
  Product1 : Product
  Trigonometric Function : Trigonometry
  Trigonometric Function1 : Trigonometry  Operator=cos
  C1 : Outport
  C2 : Outport  Port=2
  wires:
  Trigonometric Function/1 -> -C+S/2, C+S/2
  Trigonometric Function1/1 -> C+S/1, -C+S/1
  "psi "/1 -> Trigonometric Function/1, Trigonometric Function1/1
  torque/1 -> Product1/1, Product/1
  C+S/1 -> Product/2
  Product/1 -> C1/1
  Product1/1 -> C2/1
  -C+S/1 -> Product1/2

== system kinematic_control/feedback_w/mRw ==
  X_dot : Inport
  Y_dot : Inport  Port=2
  PHI : Inport  Port=3
  Add : Sum
  Add1 : Sum  Inputs=-+
  Trigonometric Function : Trigonometry
  Trigonometric Function1 : Trigonometry  Operator=cos
  xcos : Product
  xsin : Product
  ycos : Product
  ysin : Product
  xm_dot : Outport
  ym_dot : Outport  Port=2
  wires:
  PHI/1 -> Trigonometric Function1/1, Trigonometric Function/1
  X_dot/1 -> xcos/1, xsin/1
  Trigonometric Function/1 -> xsin/2, ysin/2
  Trigonometric Function1/1 -> ycos/2, xcos/2
  Y_dot/1 -> ycos/1, ysin/1
  Add1/1 -> ym_dot/1
  Add/1 -> xm_dot/1
  xcos/1 -> Add/1
  ysin/1 -> Add/2
  xsin/1 -> Add1/1
  ycos/1 -> Add1/2

== system kinematic_control/Kinematic_control/Vc_to_wc/mRw ==
  X_dot : Inport
  Y_dot : Inport  Port=2
  PHI : Inport  Port=3
  Add : Sum
  Add1 : Sum  Inputs=-+
  Trigonometric Function : Trigonometry
  Trigonometric Function1 : Trigonometry  Operator=cos
  xcos : Product
  xsin : Product
  ycos : Product
  ysin : Product
  xm_dot : Outport
  ym_dot : Outport  Port=2
  wires:
  PHI/1 -> Trigonometric Function1/1, Trigonometric Function/1
  X_dot/1 -> xcos/1, xsin/1
  Trigonometric Function/1 -> xsin/2, ysin/2
  Trigonometric Function1/1 -> ycos/2, xcos/2
  Y_dot/1 -> ycos/1, ysin/1
  Add1/1 -> ym_dot/1
  Add/1 -> xm_dot/1
  xcos/1 -> Add/1
  ysin/1 -> Add/2
  xsin/1 -> Add1/1
  ycos/1 -> Add1/2

== matlab function kinematic_control/Path_Planning/T_curve_XY  ==
  settings: updateMethod=DISCRETE  sampleTime=0.001
  data: A data_store_memory; PCmd_X_output output; Vcmd_X_output output; PCmd_Y_output output; Vcmd_Y_output output; Final_X input; TEST output; Final_X_pos data_store_memory; Vcmd_X data_store_memory; Accel_sign_X data_store_memory; Need_Dis_X data_store_memory; Need_Dis_X_Buff data_store_memory; DeAccel_X data_store_memory; Cmd_X data_store_memory; Final_Y input; Vcmd_Y data_store_memory; Final_Y_pos data_store_memory; Accel_sign_Y data_store_memory; Need_Dis_Y data_store_memory; Need_Dis_Y_Buff data_store_memory; DeAccel_Y data_store_memory; Cmd_Y data_store_memory
function [PCmd_X_output,Vcmd_X_output,PCmd_Y_output,Vcmd_Y_output,TEST]    = fcn(Final_X,Final_Y)

%==== Ver 2 =====
global A;
global Final_X_pos;
global Final_Y_pos;
global Vcmd_X;
global Vcmd_Y;
global Accel_sign_X;
global Accel_sign_Y;
global Need_Dis_X;
global Need_Dis_Y;
global Need_Dis_X_Buff;
global Need_Dis_Y_Buff;
global DeAccel_X;
global DeAccel_Y;
global Cmd_X;
global Cmd_Y;

%===== Parameter=====
Max_Accel = 1;
Max_Velocity = 2;
Pos_Standard = 0.1;
dt = 0.001;

%=== CHECK Final Change? ===
if(Final_X ~= Final_X_pos)
    Need_Dis_X = Final_X - Cmd_X;
    Need_Dis_X_Buff =0;
    DeAccel_X =0;
    
    %=== Direction Check ===
	if (Need_Dis_X >0)
        Accel_sign_X =  1;
	elseif (Need_Dis_X <0)
		Accel_sign_X = -1;
	else
		Accel_sign_X =  0;
	end
end

if(Final_Y ~= Final_Y_pos)
    Need_Dis_Y = Final_Y - Cmd_Y;
    Need_Dis_Y_Buff =0;
    DeAccel_Y =0;
    
    %=== Direction Check ===
	if (Need_Dis_Y >0)
        Accel_sign_Y =  1;
	elseif (Need_Dis_Y <0)
		Accel_sign_Y = -1;
	else
		Accel_sign_Y =  0;
	end
end

%===== Max Velocity Check =====
if( (abs(Need_Dis_X_Buff - Need_Dis_X ) > Pos_Standard) && (abs(Need_Dis_Y_Buff - Need_Dis_Y ) > Pos_Standard))
    Max_Velocity = 1.3;
else
    Max_Velocity = 2;
end



Detime_Y = abs(Vcmd_Y/Max_Accel);     
Detime_X = abs(Vcmd_X/Max_Accel);

%===== DeAccel Cehck =====
%===== X =====
     Buff = Need_Dis_X_Buff + Vcmd_X*Detime_X + 1/2*(-1*Accel_sign_X*Max_Accel)*Detime_X*Detime_X;
    
    if((Buff>Need_Dis_X) && (Accel_sign_X==1))
        DeAccel_X = 1;
    elseif ((Buff<Need_Dis_X) && (Accel_sign_X==-1))
        DeAccel_X = 1;
    else
        DeAccel_X = 0;
    end
%===== Y =====    
         Buff = Need_Dis_Y_Buff + Vcmd_Y*Detime_Y + 1/2*(-1*Accel_sign_Y*Max_Accel)*Detime_Y*Detime_Y;
    
    if((Buff>Need_Dis_Y) && (Accel_sign_Y==1))
        DeAccel_Y = 1;
    elseif ((Buff<Need_Dis_Y) && (Accel_sign_Y==-1))
        DeAccel_Y = 1;
    else
        DeAccel_Y = 0;
    end
    
%===== Vel Cal =====
%===== X =====
if(DeAccel_X ==0)
    Vcmd_X = Vcmd_X + Accel_sign_X * Max_Accel*dt;
elseif(DeAccel_X ==1) 
    Vcmd_X = Vcmd_X - Accel_sign_X * Max_Accel*dt;
    Buff = Vcmd_X *Accel_sign_X;
    if(Buff<0)
    Vcmd_X = 0;
    end
end
%===== Y =====
if(DeAccel_Y ==0)
    Vcmd_Y = Vcmd_Y + Accel_sign_Y * Max_Accel*dt;
elseif(DeAccel_Y ==1) 
    Vcmd_Y = Vcmd_Y - Accel_sign_Y * Max_Accel*dt;
    Buff = Vcmd_Y *Accel_sign_Y;
    if(Buff<0)
    Vcmd_Y = 0;
    end
end

%===== Max Vel Check =====
%=== X ===
if(Vcmd_X > Max_Velocity)
    Vcmd_X = Max_Velocity;
elseif (Vcmd_X < -Max_Velocity)
    Vcmd_X = -Max_Velocity;
end
%=== Y ===
if(Vcmd_Y > Max_Velocity)
    Vcmd_Y = Max_Velocity;
elseif (Vcmd_Y < -Max_Velocity)
    Vcmd_Y = -Max_Velocity;
end


Cmd_X = Cmd_X + Vcmd_X * dt;
Cmd_Y = Cmd_Y + Vcmd_Y * dt;

Need_Dis_X_Buff = Need_Dis_X_Buff + Vcmd_X*dt;
Need_Dis_Y_Buff = Need_Dis_Y_Buff + Vcmd_Y*dt;

Final_X_pos = Final_X;
Final_Y_pos = Final_Y;

%===== Output =====
PCmd_X_output  = Cmd_X;
PCmd_Y_output  = Cmd_Y;

Vcmd_X_output = Vcmd_X;
Vcmd_Y_output = Vcmd_Y;

A = A+1;
TEST =A;

== matlab function kinematic_control/Path_Planning/T_curve_phi/T_curve ==
  settings: updateMethod=DISCRETE  sampleTime=0.001
  data: A data_store_memory; Cmd_phi_output output; Vcmd_phi_output output; Final_phi input; TEST output; Final_phi_pos data_store_memory; Vcmd_phi data_store_memory; Accel_sign_phi data_store_memory; Need_Dis_phi data_store_memory; Need_Dis_phi_Buff data_store_memory; DeAccel_phi data_store_memory; Cmd_phi data_store_memory
function [Cmd_phi_output,Vcmd_phi_output,TEST]    = fcn(Final_phi)

%==== Ver 2 =====

global A;
global Final_phi_pos;
global Vcmd_phi;
global Accel_sign_phi;
global Need_Dis_phi;
global Need_Dis_phi_Buff;
global DeAccel_phi;
global Cmd_phi;

%===== Parameter=====
Max_Accel = pi/4;
Max_Velocity = pi/4;
Pos_Standard = 0.1;
dt = 0.001;

%=== CHECK Final Change? ===
if(Final_phi ~= Final_phi_pos)
    Need_Dis_phi = Final_phi - Cmd_phi;
    Need_Dis_phi_Buff =0;
    DeAccel_phi =0;
    
    %=== Direction Check ===
	if (Need_Dis_phi >0)
        Accel_sign_phi =  1;
	elseif (Need_Dis_phi <0)
		Accel_sign_phi = -1;
	else
		Accel_sign_phi =  0;
	end
end
    
Detime_phi = abs(Vcmd_phi/Max_Accel);

%===== DeAccel Cehck =====
     Buff = Need_Dis_phi_Buff + Vcmd_phi*Detime_phi + 1/2*(-1*Accel_sign_phi*Max_Accel)*Detime_phi*Detime_phi;
    
    if((Buff>Need_Dis_phi) && (Accel_sign_phi==1))
        DeAccel_phi = 1;
    elseif ((Buff<Need_Dis_phi) && (Accel_sign_phi==-1))
        DeAccel_phi = 1;
    else
        DeAccel_phi = 0;
    end
    
%===== Vel Cal =====
if(DeAccel_phi ==0)
    Vcmd_phi = Vcmd_phi + Accel_sign_phi * Max_Accel*dt;
elseif(DeAccel_phi ==1) 
    Vcmd_phi = Vcmd_phi - Accel_sign_phi * Max_Accel*dt;
    Buff = Vcmd_phi *Accel_sign_phi;
    if(Buff<0)
    Vcmd_phi = 0;
    end
end

%===== Max Vel Check =====

if(Vcmd_phi > Max_Velocity)
    Vcmd_phi = Max_Velocity;
elseif (Vcmd_phi < -Max_Velocity)
    Vcmd_phi = -Max_Velocity;
end


Cmd_phi = Cmd_phi + Vcmd_phi * dt;
Need_Dis_phi_Buff = Need_Dis_phi_Buff + Vcmd_phi*dt;
Final_phi_pos = Final_phi;

%===== Output =====
Cmd_phi_output  = Cmd_phi ;
Vcmd_phi_output = Vcmd_phi;

A = A+1;
TEST =A;
